simulink model "A6_Frequenzgang_PZ"  (R2017b)
settings: Solver=ode45  StartTime=0.0  StopTime=10  MaxStep=1E-3  RelTol=1e-3  EnableMultiTasking=on
undefined symbols (not defined in the file or in its folder): j
settings Model: Creator=jbaur  LastModifiedBy=jbaur
settings DataIOCC: ExternalInput=X1  SaveFormat=StructureWithTime  SignalLoggingName=sigsOut
settings OptimizationCC: ExpressionDepthLimit=2147483647  InitFltsAndDblsToZero=on  LifeSpan=inf
settings DebuggingCC: SaveWithParameterizedLinksMsg=none  SignalResolutionControl=TryResolveAllWithWarning  MultiTaskDSMMsg=warning  MultiTaskCondExecSysMsg=none  StateNameClashWarn=warning  SFUnexpectedBacktrackingDiag=warning  SFNoUnconditionalDefaultTransitionDiag=warning  SFExecutionAtInitializationDiag=none
settings HardwareCC: ProdBitPerPointer=32  ProdBitPerSizeT=32  ProdBitPerPtrDiffT=32  ProdLargestAtomicFloat=None  ProdIntDivRoundTo=Undefined  ProdEndianess=Unspecified  ProdWordSize=32  ProdHWDeviceType=32-bit Generic  TargetUnknown=on
settings ModelReferenceCC: PropagateSignalLabelsOutOfModel=off
settings CodeAppCC: StateflowObjectComments=on
settings GRTTargetCC: TargetFcnLib=ansi_tfl_tmw.mat  TargetLangStandard=C89/C90 (ANSI)  ModelReferenceCompliant=off  GeneratePreprocessorConditionals=Disable all  CombineOutputUpdateFcns=off  MatFileLogging=off  GRTInterface=on
settings ConfigComp: CovMetricSettings=dw  CovHtmlReporting=on  CovSaveCumulativeToWorkspaceVar=on  CovSaveSingleToWorkspaceVar=on  CovExternalEMLEnable=off  CovSFcnEnable=off

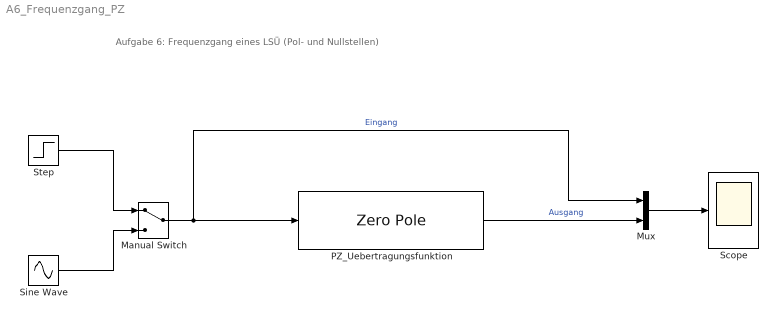
== system A6_Frequenzgang_PZ ==
  note: Aufgabe 6: Frequenzgang eines LSÜ (Pol- und Nullstellen)
  Manual Switch : ManualSwitch
  Mux : Mux  Inputs=2
  PZ_Uebertragungsfunktion : ZeroPole  Poles=[-1+2*j -1-2*j]
  Scope : Scope
  Sine Wave : Sin  SampleTime=0
  Step : Step  Time=0  SampleTime=0
  wires:
  Mux/1 -> Scope/1
  Step/1 -> Manual Switch/1
  Sine Wave/1 -> Manual Switch/2
  PZ_Uebertragungsfunktion/1 -> Mux/2  "Ausgang"
  Manual Switch/1 -> Mux/1, PZ_Uebertragungsfunktion/1  "Eingang"
